simulink model "Decimator_SSR"  (R2023b)
settings: Solver=VariableStepAuto  StartTime=0.0  StopTime=6000*(1/Fclk)  RelTol=1e-3
PreLoadFcn:
  | startup
undefined symbols (not defined in the file): Fclk, SSRin
libraries: hdlBasic x10, hdlSSR x6, dspsrcs4 x1, vmcUtilities x1
settings Model: Creator=Jakub  LastModifiedBy=andre

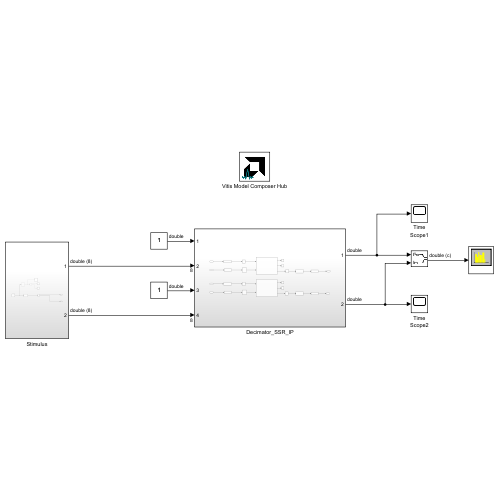
[thumbnail: Simulink's stored preview of the top-level diagram]
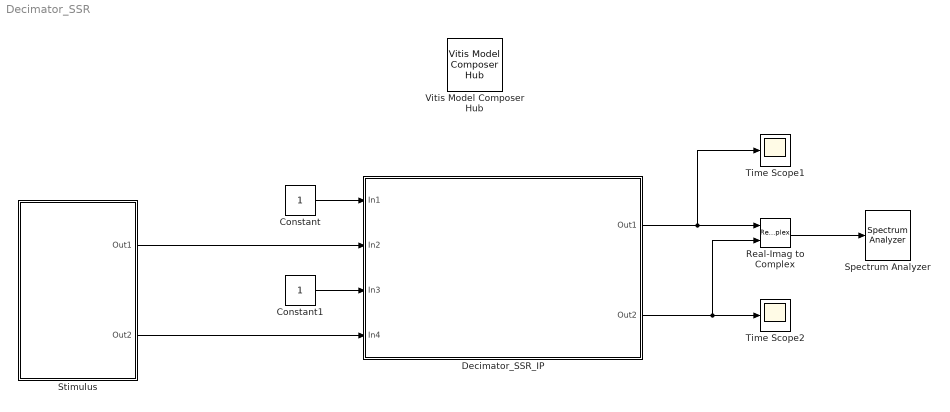
== system Decimator_SSR ==
  Constant : Constant
  Constant1 : Constant
  Decimator_SSR_IP : Subsystem
  Real-Imag to Complex : RealImagToComplex
  Spectrum Analyzer : SpectrumAnalyzer  WindowPosition=[364.000000,73.000000,800.000000,500.000000,]  Visible=on  ScopeFrameLocation=window  Span=64000000  StartFrequency=-32000000  StopFrequency=32000000  YLimits=[-99.64753716,-15.58397496]  SelectedToolstripTab=spectrumAnalyzerToolstrip.measurementsTab
  Stimulus : Subsystem
  Time Scope1 : Scope
  Time Scope2 : Scope
  Vitis Model Composer Hub : vmcUtilities/Vitis Model Composer Hub  Tag=genX  CodeGeneration=off  SubsystemName=Decimator_SSR_IP  DUTSubsystemName=Decimator_SSR_IP  CompilationType=HDLCompilation  ExportTypeV2=HDL Netlist  TargetDirectory=./netlist\ip\Decimator_SSR_IP\src  exportDesign=on  analyzeDesign=off  validateDesignOnHw=off  ExportType=HDL  IpVendor=xilinx.com  IpLibrary=hls  IpVersion=1.0  IpHWLanguage=Verilog  AieCompilerOptions={}  AieSimulatorOptions={}  CreateTestbench=off  TestbenchStackSize=10  RunRtlSim=off  RunCSim=off  RunAieSim=off  AieSimTimeout=50000  RunAieSimProfiling=off  LaunchVitisAnalyzer=off  PlotOutput=off  RunX86Sim=off  X86SimTimeout=10  GenHwImage=off  GenLibadfXo=on  GenHwValidationCode=off  PlatformType=Not Specified  HwSystemType=Baremetal  HwValidationTarget=hw  ProjDevice=Zynq UltraScale+ ZCU111 Evaluation Platform (xczu28dr-ffvg1517-2-e)  ProjDevicePart=xczu28dr-ffvg1517-2-e  SamplePeriod=-1  ClockFrequency=200  DataPathParallelism=1  xilinxfamily=zynquplusRFSOC  part=xczu28dr  speed=-2-e  package=ffvg1517  directory=./netlist\ip\Decimator_SSR_IP\src  testbench=off  incr_netlist=off  synthesis_tool=Vivado  clock_wrapper=Clock Enables  dbl_ovrd=According to Block Masks  dcm_input_clock_period=10  sysclk_period=(1/Fclk)*(1e6)  simulink_period=1/Fclk  eval_field=0  IPInfoJsonString="{\"HDLSubsystem\":{\"SubsystemName\":\"Decimator_SSR_IP\",\"IPName\":\"Subsystem\",\"IPLibrary\":\"VMC\",\"IPVendor\":\"User Company\",\"IPVersion\":\"1.0\",\"TargetDirectory\":\"./netlist\",\"SubsystemDir\":\"./netlist\\\\ip\\\\Decimator_SSR_IP\"},\"SubsystemTag\":\"HDLNode\"}"  LogFileName=''  NThreads=4
  wires:
  Constant1/1 -> Decimator_SSR_IP/3(In3)
  Constant/1 -> Decimator_SSR_IP/1(In1)
  Stimulus/1(Out1) -> Decimator_SSR_IP/2(In2)
  Stimulus/2(Out2) -> Decimator_SSR_IP/4(In4)
  Decimator_SSR_IP/1(Out1) -> Time Scope1/1, Real-Imag to Complex/1
  Decimator_SSR_IP/2(Out2) -> Time Scope2/1, Real-Imag to Complex/2
  Real-Imag to Complex/1 -> Spectrum Analyzer/1

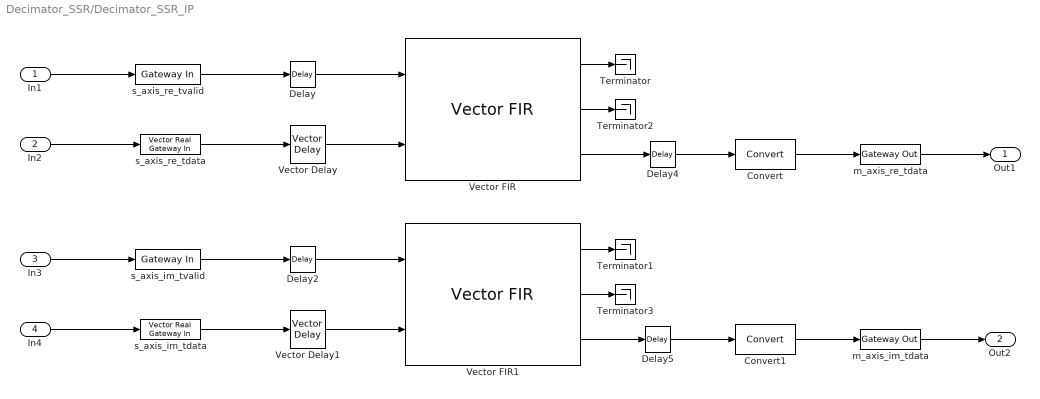
== system Decimator_SSR/Decimator_SSR_IP ==
  In1 : Inport
  In2 : Inport  Port=2
  In3 : Inport  Port=3
  In4 : Inport  Port=4
  Convert : hdlBasic/Convert  gui_display_data_type=Fixed-point  arith_type=Signed (2's comp)  n_bits=16  bin_pt=15  float_type=Single  exp_bits=8  fraction_bits=24  quantization=Truncate  overflow=Saturate  en=off  latency=1  pipeline=off  XmcBlockStatus=1  maskContainerNames=group2  block_type=convert  block_config=sysgen:Convert_config  block_width=595  block_height=885
  Convert1 : hdlBasic/Convert  gui_display_data_type=Fixed-point  arith_type=Signed (2's comp)  n_bits=16  bin_pt=15  float_type=Single  exp_bits=8  fraction_bits=24  quantization=Truncate  overflow=Saturate  en=off  latency=1  pipeline=off  XmcBlockStatus=1  maskContainerNames=group2  block_type=convert  block_config=sysgen:Convert_config  block_width=595  block_height=885
  Delay{,2,4..5} (4 alike) : hdlBasic/Delay  rst=off  en=off  latency=1  reg_retiming=off  XmcBlockStatus=1  maskContainerNames=group1  block_type=delay  block_config=sysgen:Delay_config
  Terminator{,1..3} (4 alike) : Terminator
  Vector Delay : hdlSSR/Vector Delay  rst=off  en=off  vectorize_en=off  sg_latency=1  sg_ssr=SSRin  reg_retiming=off  block_type=delay_ssr  XmcBlockStatus=1  sg_ssr_prev=8  maskContainerNames=group1
  Vector Delay1 : hdlSSR/Vector Delay  rst=off  en=off  vectorize_en=off  sg_latency=1  sg_ssr=SSRin  reg_retiming=off  block_type=delay_ssr  XmcBlockStatus=1  sg_ssr_prev=8  maskContainerNames=group1
  Vector FIR : hdlSSR/Vector FIR  coefficientvector=W  coefficient_sets=1  coefficient_reload=off  filter_type=Decimation  rate_change_type=Integer  interpolation_rate=1  decimation_rate=8  zero_pack_factor=1  sg_ssr=SSRin  coefficient_sign=Signed  quantization=Quantize_Only  coefficient_width=16  bestprecision=on  coefficient_fractional_bits=15  coefficient_structure=Inferred  output_rounding_mode=Full_Precision  output_width=16  filter_architecture=Transpose_Multiply_Accumulate  optimization_goal=Speed  optimization_list='None'  data_buffer_type=Automatic  coefficient_buffer_type=Automatic  input_buffer_type=Automatic  output_buffer_type=Automatic  preference_for_other_storage=Automatic  multi_column_support=Automatic  columnconfig='1'  inter_column_pipe_length=4  m_data_has_tready=off  has_aclken=off  has_aresetn=off  reset_data_vector=on  simulation_type=hybrid_sim  simulation_model=sysgen:xfirv7_2_cmodel  data_path_portlist={ 's_axis_data_tdata', 'm_axis_data_tdata' }  passband_min=0.0  passband_max=0.5  stopband_min=0.5  stopband_max=1.0  filter_selection=1  gui_behaviour=Sysgen_GUI  data_sign=Signed  data_width=16  data_fractional_bits=0  data_tuser_width=1  wrapper_available=true  ip_wrap_arbitrary_binary_point=true  ip_name=FIR Compiler  ip_version=7.2  dsptool_ready=true  ipcore_usecache=true  ipcore_useipmodelcache=true  port_translation_map={ 'aclken' => 'en', 'aresetn' => 'rst' }  run_core_at_system_period=true  ipcore_xco_need_fpga_part=true  ipcore_fpga_part=[]  block_type=fir_compiler_v7_2_ssr  decimation_prev=8  interpolation_prev=1  coeffsets_prev=1  filter_prev=Decimation  channel_sequence=Basic  number_channels=1  pattern_list='P4-0,P4-1,P4-2,P4-3,P4-4'  number_paths=1  data_has_tlast=Not_Required  s_data_has_fifo=off  s_data_has_tuser=Not_Required  m_data_has_tuser=Not_Required  s_config_sync_mode=On_Vector  s_config_method=Single  num_reload_slots=1  XmcBlockStatus=1  sg_ssr_prev=8  maskContainerNames=group10  block_width=657
      settings: block_version=1.0
  Vector FIR1 : hdlSSR/Vector FIR  coefficientvector=W  coefficient_sets=1  coefficient_reload=off  filter_type=Decimation  rate_change_type=Integer  interpolation_rate=1  decimation_rate=8  zero_pack_factor=1  sg_ssr=SSRin  coefficient_sign=Signed  quantization=Quantize_Only  coefficient_width=16  bestprecision=on  coefficient_fractional_bits=15  coefficient_structure=Inferred  output_rounding_mode=Full_Precision  output_width=16  filter_architecture=Transpose_Multiply_Accumulate  optimization_goal=Speed  optimization_list='None'  data_buffer_type=Automatic  coefficient_buffer_type=Automatic  input_buffer_type=Automatic  output_buffer_type=Automatic  preference_for_other_storage=Automatic  multi_column_support=Automatic  columnconfig='1'  inter_column_pipe_length=4  m_data_has_tready=off  has_aclken=off  has_aresetn=off  reset_data_vector=on  simulation_type=hybrid_sim  simulation_model=sysgen:xfirv7_2_cmodel  data_path_portlist={ 's_axis_data_tdata', 'm_axis_data_tdata' }  passband_min=0.0  passband_max=0.5  stopband_min=0.5  stopband_max=1.0  filter_selection=1  gui_behaviour=Sysgen_GUI  data_sign=Signed  data_width=16  data_fractional_bits=0  data_tuser_width=1  wrapper_available=true  ip_wrap_arbitrary_binary_point=true  ip_name=FIR Compiler  ip_version=7.2  dsptool_ready=true  ipcore_usecache=true  ipcore_useipmodelcache=true  port_translation_map={ 'aclken' => 'en', 'aresetn' => 'rst' }  run_core_at_system_period=true  ipcore_xco_need_fpga_part=true  ipcore_fpga_part=[]  block_type=fir_compiler_v7_2_ssr  decimation_prev=8  interpolation_prev=1  coeffsets_prev=1  filter_prev=Decimation  channel_sequence=Basic  number_channels=1  pattern_list='P4-0,P4-1,P4-2,P4-3,P4-4'  number_paths=1  data_has_tlast=Not_Required  s_data_has_fifo=off  s_data_has_tuser=Not_Required  m_data_has_tuser=Not_Required  s_config_sync_mode=On_Vector  s_config_method=Single  num_reload_slots=1  XmcBlockStatus=1  sg_ssr_prev=8  maskContainerNames=group10  block_width=657
      settings: block_version=1.0
  m_axis_im_tdata : hdlBasic/Gateway Out  inherit_from_input=off  hdl_port=on  rows=1  columns=1  UseAsDAC=off  DACChannel='1'  interface=None  automatic_assignment=on  address_offset=hex2dec('00')  intf_name=''  intf_description=''  timing_constraint=None  locs_specified=off  LOCs={}  io_standard={}  XmcBlockStatus=1  maskContainerNames=group4  block_type=gatewayout  block_config=sysgen:gateway_out_config  block_width_w=590  block_height_w=620  block_width=620  block_height=750
  m_axis_re_tdata : hdlBasic/Gateway Out  inherit_from_input=off  hdl_port=on  rows=1  columns=1  UseAsDAC=off  DACChannel='1'  interface=None  automatic_assignment=on  address_offset=hex2dec('00')  intf_name=''  intf_description=''  timing_constraint=None  locs_specified=off  LOCs={}  io_standard={}  XmcBlockStatus=1  maskContainerNames=group4  block_type=gatewayout  block_config=sysgen:gateway_out_config  block_width_w=590  block_height_w=620  block_width=620  block_height=750
  s_axis_im_tdata : hdlSSR/Vector Real Gateway In  gui_display_data_type=Fixed-point  arith_type=Signed (2's comp)  n_bits=16  bin_pt=15  preci_type=Single  exp_width=8  frac_width=24  quantization="Round  (unbiased: +/- Inf)"  overflow=Saturate  period=1/Fclk  sg_ssr=8  UseAsADC=off  ADCChannel='1'  interface=None  automatic_assignment=on  address_offset=hex2dec('00')  intf_name=''  intf_description=''  default_value=0  timing_constraint=None  locs_specified=off  LOCs={}  io_standard={}  inherit_from_input=off  hdl_port=on  interface_prev=1  block_type=realgatewayin_ssr  XmcBlockStatus=1  sg_ssr_prev=8  maskContainerNames=group4  block_width_w=590  block_height_w=670  block_width=640  block_height=850
  s_axis_im_tvalid : hdlBasic/Gateway In  gui_display_data_type=Boolean  arith_type=Boolean  n_bits=16  bin_pt=14  preci_type=Single  exp_width=8  frac_width=24  rows=1  columns=1  quantization="Round  (unbiased: +/- Inf)"  overflow=Saturate  period=1/Fclk  UseAsADC=off  ADCChannel='1'  interface=None  automatic_assignment=on  address_offset=hex2dec('00')  intf_name=''  intf_description=''  default_value=0  timing_constraint=None  locs_specified=off  LOCs={}  io_standard={}  inherit_from_input=off  hdl_port=on  XmcBlockStatus=1  maskContainerNames=group4  block_type=gatewayin  block_config=sysgen:gateway_in_config  block_width_w=590  block_height_w=620  block_width=640  block_height=850
  s_axis_re_tdata : hdlSSR/Vector Real Gateway In  gui_display_data_type=Fixed-point  arith_type=Signed (2's comp)  n_bits=16  bin_pt=15  preci_type=Single  exp_width=8  frac_width=24  quantization="Round  (unbiased: +/- Inf)"  overflow=Saturate  period=1/Fclk  sg_ssr=8  UseAsADC=off  ADCChannel='1'  interface=None  automatic_assignment=on  address_offset=hex2dec('00')  intf_name=''  intf_description=''  default_value=0  timing_constraint=None  locs_specified=off  LOCs={}  io_standard={}  inherit_from_input=off  hdl_port=on  interface_prev=1  block_type=realgatewayin_ssr  XmcBlockStatus=1  sg_ssr_prev=8  maskContainerNames=group4  block_width_w=590  block_height_w=670  block_width=640  block_height=850
  s_axis_re_tvalid : hdlBasic/Gateway In  gui_display_data_type=Boolean  arith_type=Boolean  n_bits=16  bin_pt=14  preci_type=Single  exp_width=8  frac_width=24  rows=1  columns=1  quantization="Round  (unbiased: +/- Inf)"  overflow=Saturate  period=1/Fclk  UseAsADC=off  ADCChannel='1'  interface=None  automatic_assignment=on  address_offset=hex2dec('00')  intf_name=''  intf_description=''  default_value=0  timing_constraint=None  locs_specified=off  LOCs={}  io_standard={}  inherit_from_input=off  hdl_port=on  XmcBlockStatus=1  maskContainerNames=group4  block_type=gatewayin  block_config=sysgen:gateway_in_config  block_width_w=590  block_height_w=620  block_width=640  block_height=850
  Out1 : Outport
  Out2 : Outport  Port=2
  wires:
  s_axis_re_tdata/1 -> Vector Delay/1
  Vector FIR1/2 -> Terminator3/1
  s_axis_im_tdata/1 -> Vector Delay1/1
  Vector FIR/1 -> Terminator/1
  Vector FIR1/1 -> Terminator1/1
  Vector FIR/2 -> Terminator2/1
  In2/1 -> s_axis_re_tdata/1
  s_axis_re_tvalid/1 -> Delay/1
  s_axis_im_tvalid/1 -> Delay2/1
  In4/1 -> s_axis_im_tdata/1
  m_axis_im_tdata/1 -> Out2/1
  In1/1 -> s_axis_re_tvalid/1
  m_axis_re_tdata/1 -> Out1/1
  In3/1 -> s_axis_im_tvalid/1
  Vector FIR1/3 -> Delay5/1
  Vector FIR/3 -> Delay4/1
  Convert/1 -> m_axis_re_tdata/1
  Convert1/1 -> m_axis_im_tdata/1
  Delay/1 -> Vector FIR/1
  Vector Delay/1 -> Vector FIR/2
  Delay2/1 -> Vector FIR1/1
  Vector Delay1/1 -> Vector FIR1/2
  Delay5/1 -> Convert1/1
  Delay4/1 -> Convert/1

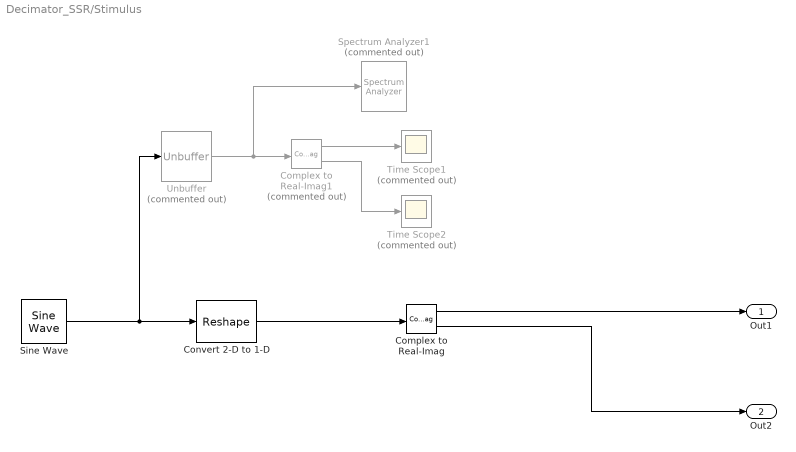
== system Decimator_SSR/Stimulus ==
  Complex to Real-Imag : ComplexToRealImag
  Complex to Real-Imag1 : ComplexToRealImag  Commented=on
  Convert 2-D to 1-D : Reshape
  Sine Wave : dspsrcs4/Sine Wave  Amplitude=0.9  Frequency=4e6  Phase=0  SampleMode=Discrete  OutComplex=Complex  CompMethod=Trigonometric fcn  TableSize=Speed  SampleTime=1/(Fclk*SSRin)  SamplesPerFrame=8  ResetState=Restart at time zero  OutputFrames=off  dataType=double  wordLen=16  udDataType=sfix(16)  fracBitsMode=Best precision  numFracBits=15  OutDataTypeStr=double  LastOutDataTypeStr=double
  Spectrum Analyzer1 : SpectrumAnalyzer  Commented=on  WindowPosition=[482.000000,-114.000000,799.000000,500.000000,]  ScopeFrameLocation=window  Span=512000000  StartFrequency=-256000000  StopFrequency=256000000  YLimits=[-76.70327565,40.8002869]  SelectedToolstripTab=spectrumAnalyzerToolstrip.measurementsTab
  Time Scope1 : Scope  Commented=on
  Time Scope2 : Scope  Commented=on
  Unbuffer : Unbuffer  Commented=on
  Out1 : Outport
  Out2 : Outport  Port=2
  wires:
  Sine Wave/1 -> Unbuffer/1, Convert 2-D to 1-D/1
  Convert 2-D to 1-D/1 -> Complex to Real-Imag/1
  Complex to Real-Imag/1 -> Out1/1
  Complex to Real-Imag/2 -> Out2/1
  Unbuffer/1 -> Complex to Real-Imag1/1, Spectrum Analyzer1/1
  Complex to Real-Imag1/1 -> Time Scope1/1
  Complex to Real-Imag1/2 -> Time Scope2/1
